simulink model "FAULTANALYSIS"  (R2022b)
settings: Solver=VariableStepAuto  StartTime=0.0  StopTime=10.0  RelTol=1e-3
undefined symbols (not defined in the file or in its folder): D1, Delta
libraries: spsRMSLib x3, simulink_extras x3, spsThreePhaseVIMeasurementLib x1, spsThreePhaseBreakerLib x1, spsThreePhaseTransformerTwoWindingsLib x1, spsThreePhaseParallelRLCLoadLib x1, spsThreePhaseFaultLib x1, spsThreePhaseSourceLib x1, spspowerguiLib x1
settings Model: Creator=dewan  LastModifiedBy=dewan

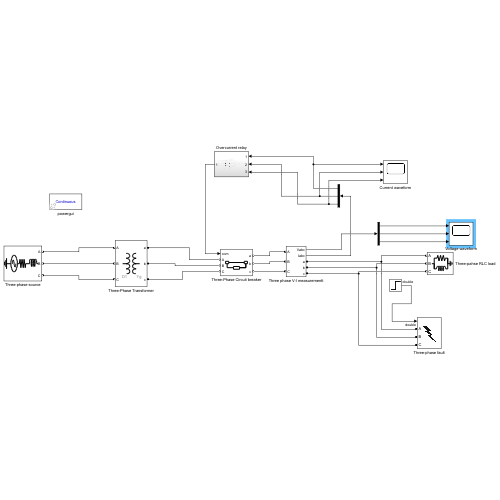
[thumbnail: Simulink's stored preview of the top-level diagram]
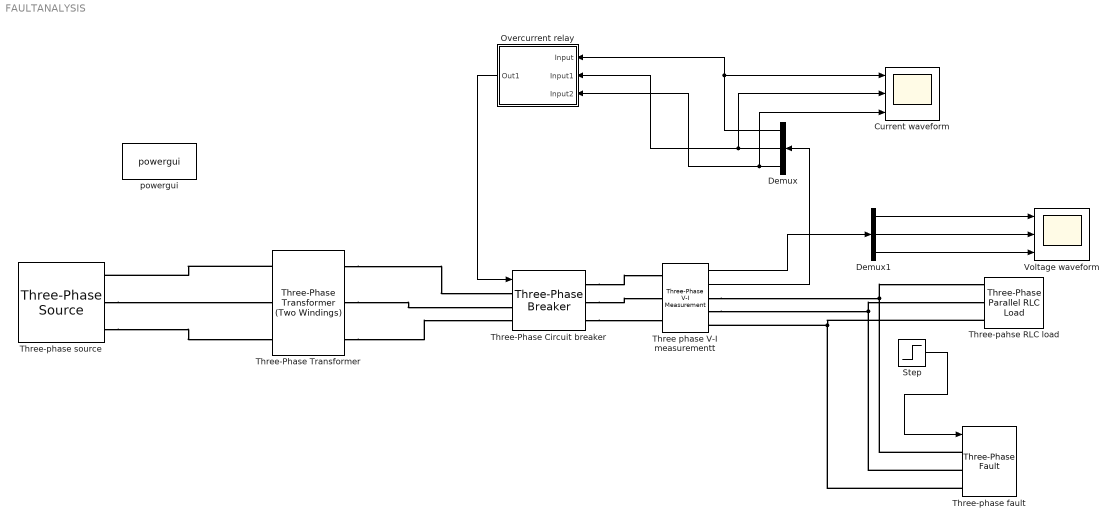
== system FAULTANALYSIS ==
  Current waveform : Scope  NumInputPorts=3
  Demux : Demux  Outputs=3
  Demux1 : Demux  Outputs=3
  Overcurrent relay : Subsystem
  Step : Step  Time=0.1  SampleTime=0
  Three phase V-I measurementt : spsThreePhaseVIMeasurementLib/Three-Phase V-I Measurement  VoltageMeasurement=phase-to-ground  SetLabelV=off  LabelV=Vabc  Vpu=off  VpuLL=off  CurrentMeasurement=yes  SetLabelI=off  LabelI=Iabc  Ipu=off  Pbase=100e6  Vbase=500e3  OutputType=Complex  PhasorSimulation=off  PSBequivalent=0
  Three-Phase Circuit breaker : spsThreePhaseBreakerLib/Three-Phase Breaker  InitialState=closed  SwitchA=on  SwitchB=on  SwitchC=on  SwitchTimes="[1/50  5/50]"  External=on  BreakerResistance=0.01  SnubberResistance=1e6  SnubberCapacitance=inf  Measurements=None
  "Three-Phase Transformer " : spsThreePhaseTransformerTwoWindingsLib/Three-Phase Transformer (Two Windings)  Winding1Connection=Delta (D1)  Winding2Connection=Yg  CoreType=Three single-phase transformers  SetSaturation=off  Hysteresis=off  DataFile='hysteresis'  SetInitialFlux=off  Measurements=None  UNITS=pu  NominalPower=[ 10e6 , 50 ]  Winding1=[ 11e3 , 0.002 , 0.08 ]  Winding2=[ 4.4e3 , 0.002 , 0.08 ]  Rm=500  Lm=500  L0=0.5  Saturation=[ 0,0 ; 0.0024,1.2 ; 1.0,1.52 ]  InitialFluxes=[ 0.8 , -0.8 , 0.7 ]  BreakLoop=off  DiscreteSolver=Trapezoidal iterative  DataType=off  TransfoNumber=1
  Three-pahse RLC load : spsThreePhaseParallelRLCLoadLib/Three-Phase Parallel RLC Load  LConnTagsString=A|B|C  Configuration=Y (grounded)  NominalVoltage=4.4e3  Vabc=[1e3 1e3 1e3]  Vabcp=[1e3 1e3 1e3]  NominalFrequency=50  UnbalancedPower=off  ActivePower=5e6  InductivePower=20e3  CapacitivePower=0  Pabc=[10e3 9e3 11e3]  QLabc=[100 90 110]  QCabc=[100 90 110]  Pabcp=[10e3 9e3 11e3]  QLabcp=[100 90 110]  QCabcp=[100 90 110]  Measurements=None  LoadType=constant Z
  Three-phase fault : spsThreePhaseFaultLib/Three-Phase Fault  InitialStates=0  FaultA=on  FaultB=on  FaultC=on  GroundFault=on  SwitchTimes="[1/50  5/50]"  External=on  SwitchStatus=NaN  FaultResistance=0.001  GroundResistance=0.01  SnubberResistance=1e6  SnubberCapacitance=inf  Measurements=None
  Three-phase source : spsThreePhaseSourceLib/Three-Phase Source  InternalConnection=Yg  VoltagePhases=off  Voltage=11e3  PhaseAngle=0  Voltage_phases=[25e3 25e3 25e3]/sqrt(3)  PhaseAngles_phases=[0 -120 +120]  Frequency=50  NonIdealSource=on  SpecifyImpedance=on  Resistance=0.8929  Inductance=16.58e-3  ShortCircuitLevel=20e6  BaseVoltage=11e3  XRratio=7  BusType=swing  Pref=10e3  Qref=0  Prefabc=[10e3, 10e3, 10e3]  Qrefabc=[0, 0, 0]  Qmin=-inf  Qmax=inf
  Voltage waveform : Scope  NumInputPorts=3
  powergui : spspowerguiLib/powergui  Priority=1  SimulationMode=Continuous  SampleTime=50e-6  frequency=60  Iterations=50  frequencyindice=50  Pbase=100e6  ErrMax=1e-4  UnitsV=kV  UnitsW=MW  buscounter=0  FunctionMessages=off  echomessages=off  EnableUseOfTLC=off  CurrentSourceSwitches=off  DisableSnubberDevices=off  DisableRonSwitches=off  DisableVfSwitches=off  DisplayEquations=off  AutomaticDiscreteSolvers=off  SolverType=Tustin/Backward Euler (TBE)  Interpol=off  ExternalGateDelay=off  methode=off  Ts=100  x0status=blocks  SPID=on  SwTol=0  HookPort=off  NonlinearTolerance=1e-4  nMaxIteration=100  ContinueOnMaxIteration=off  RestoreLinks=warning  ResistiveCurrentMeasurement=off  Frange=[0:2:500]  Ylog=off  Xlog=on  ShowGrid=off  save=off  variable=ZData  structure=0  ZoomFFT=off  StartTime=0.0  cycles=1  DisplayStyle=1  fundamental=60  FreqAxis=off  MaxFrequency=1000  frequencyindicesteady=1  RmsSteady=1  display=off
  wires:
  Step/1 -> Three-phase fault/1
  Demux/3 -> Overcurrent relay/3(Input2), Current waveform/3
  Demux/2 -> Current waveform/2, Overcurrent relay/2(Input1)
  Demux/1 -> Current waveform/1, Overcurrent relay/1(Input)
  Three phase V-I measurementt/2 -> Demux/1
  Three phase V-I measurementt/1 -> Demux1/1
  Demux1/3 -> Voltage waveform/3
  Demux1/2 -> Voltage waveform/2
  Demux1/1 -> Voltage waveform/1
  Overcurrent relay/1(Out1) -> Three-Phase Circuit breaker/1
  connections:
  "Three-Phase Transformer "/LConn1 -- Three-phase source/RConn1
  Three-phase source/RConn2 -- "Three-Phase Transformer "/LConn2
  Three-phase source/RConn3 -- "Three-Phase Transformer "/LConn3
  Three-pahse RLC load/LConn3 -- Three phase V-I measurementt/RConn3 -- Three-phase fault/LConn3
  Three phase V-I measurementt/RConn2 -- Three-phase fault/LConn2 -- Three-pahse RLC load/LConn2
  Three phase V-I measurementt/RConn1 -- Three-pahse RLC load/LConn1 -- Three-phase fault/LConn1
  "Three-Phase Transformer "/RConn3 -- Three-Phase Circuit breaker/LConn3
  "Three-Phase Transformer "/RConn2 -- Three-Phase Circuit breaker/LConn2
  "Three-Phase Transformer "/RConn1 -- Three-Phase Circuit breaker/LConn1
  Three-Phase Circuit breaker/RConn3 -- Three phase V-I measurementt/LConn3
  Three-Phase Circuit breaker/RConn2 -- Three phase V-I measurementt/LConn2
  Three-Phase Circuit breaker/RConn1 -- Three phase V-I measurementt/LConn1

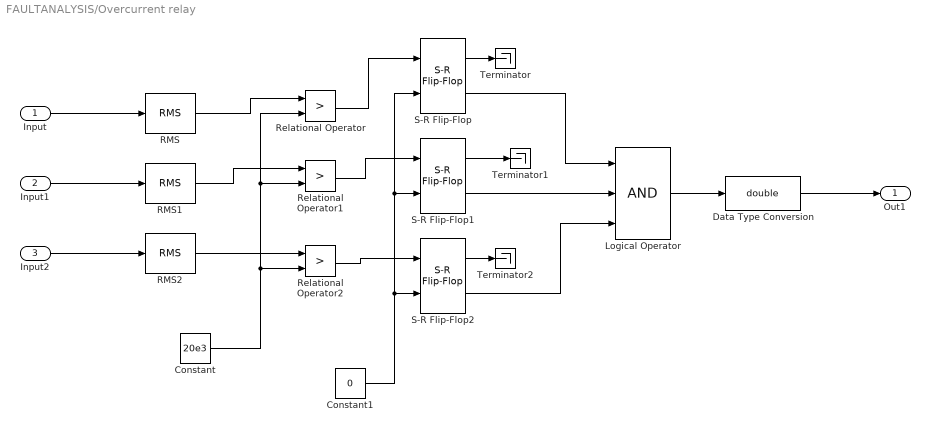
== system FAULTANALYSIS/Overcurrent relay ==
  Input : Inport
  Input1 : Inport  Port=2
  Input2 : Inport  Port=3
  Constant : Constant  Value=20e3
  Constant1 : Constant  Value=0
  Data Type Conversion : DataTypeConversion  OutDataTypeStr=double  SaturateOnIntegerOverflow=off  RndMeth=Floor
  Logical Operator : Logic  Inputs=3  AllPortsSameDT=off  OutDataTypeStr=boolean
  RMS : spsRMSLib/RMS  TrueRMS=on  Freq=50  RMSInit=0  Ts=0.001
  RMS1 : spsRMSLib/RMS  TrueRMS=on  Freq=50  RMSInit=0  Ts=0.001
  RMS2 : spsRMSLib/RMS  TrueRMS=on  Freq=50  RMSInit=0  Ts=0.001
  Relational Operator : RelationalOperator  Operator=>  OutDataTypeStr=boolean  RndMeth=Simplest  InputSameDT=off
  Relational Operator1 : RelationalOperator  Operator=>  OutDataTypeStr=boolean  RndMeth=Simplest  InputSameDT=off
  Relational Operator2 : RelationalOperator  Operator=>  OutDataTypeStr=boolean  RndMeth=Simplest  InputSameDT=off
  S-R Flip-Flop : simulink_extras/Flip Flops/S-R Flip-Flop  initial_condition=0
  S-R Flip-Flop1 : simulink_extras/Flip Flops/S-R Flip-Flop  initial_condition=0
  S-R Flip-Flop2 : simulink_extras/Flip Flops/S-R Flip-Flop  initial_condition=0
  Terminator : Terminator
  Terminator1 : Terminator
  Terminator2 : Terminator
  Out1 : Outport
  wires:
  RMS2/1 -> Relational Operator2/1
  RMS/1 -> Relational Operator/1
  Input1/1 -> RMS1/1
  S-R Flip-Flop2/1 -> Terminator2/1
  Constant/1 -> Relational Operator2/2, Relational Operator1/2, Relational Operator/2
  Logical Operator/1 -> Data Type Conversion/1
  Constant1/1 -> S-R Flip-Flop2/2, S-R Flip-Flop1/2, S-R Flip-Flop/2
  S-R Flip-Flop1/1 -> Terminator1/1
  Input/1 -> RMS/1
  S-R Flip-Flop2/2 -> Logical Operator/3
  Data Type Conversion/1 -> Out1/1
  S-R Flip-Flop/1 -> Terminator/1
  S-R Flip-Flop1/2 -> Logical Operator/2
  Relational Operator2/1 -> S-R Flip-Flop2/1
  S-R Flip-Flop/2 -> Logical Operator/1
  Relational Operator/1 -> S-R Flip-Flop/1
  Input2/1 -> RMS2/1
  RMS1/1 -> Relational Operator1/1
  Relational Operator1/1 -> S-R Flip-Flop1/1
